simulink model "Robot_puma_system"  (R2018b)
settings: Solver=ode45  StartTime=0.0  StopTime=5  FixedStep=0.01  MaxStep=0.01  RelTol=1e-3
values from neighbouring files (symbols this model uses):
  AmpSat1 = 12    [CONSTANT.m]
  BackEMF1 = (12 - 38.1*0.2)/(40*2*pi/60)    (= 1.04564797611)    [CONSTANT.m]
  BackEMF2 = 0.32    [CONSTANT.m]
  BackEMF3 = 0.00091    [CONSTANT.m]
  CtlSat1 = 1024    [CONSTANT.m]
  Elec1d = [termL, termR1]    [CONSTANT.m]
  Elec1n = 1    [CONSTANT.m]
  Elec2d = [termL, termR2]    [CONSTANT.m]
  KP = [700 0 0 0 0 0; 0 670 0 0 0 0; 0 0 650 0 0 0; 0 0 0 400*5/1.5 0 0; 0 0 0 0 540*5/1.5 0; 0 0 0 0 0 210*5/1.5]    [CONSTANT.m]
  KV = [400 0 0 0 0 0; 0 470 0 0 0 0; 0 0 550 0 0 0; 0 0 0 370*5/1.5 0 0; 0 0 0 0 60*5/1.5 0; 0 0 0 0 0 180*5/1.5]    [CONSTANT.m]
  PWM_CONV_OTHER = 1.0/1024.0    (= 0.0009765625)    [CONSTANT.m]
  Starting_Pos = [0;3.1415926/5;3.1415926/6;3.1415926/10;3.1415926/7;3.1415926/2]    [CONSTANT.m]
  TConst1 = 1.207    [CONSTANT.m]
  TConst2 = 0.5324    [CONSTANT.m]
  TConst3 = 0.089240515    [CONSTANT.m]
settings Model: SimulationMode=accelerator  Creator=zhikai  LastModifiedBy=zhikai
settings SolverCC: AlgebraicLoopSolver=LineSearch
settings DataIOCC: SaveFinalState=on  SaveCompleteFinalSimState=on  SaveState=on

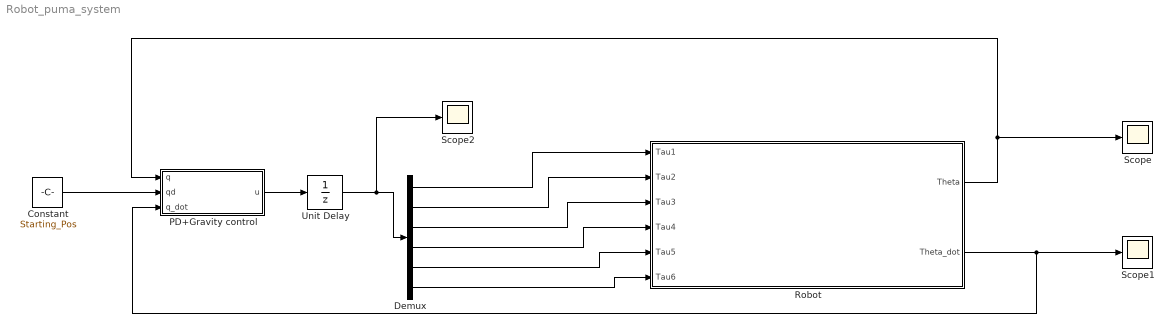
== system Robot_puma_system ==
  Constant : Constant  Value=Starting_Pos
  Demux : Demux  Outputs=6
  PD+Gravity control : Subsystem  TreatAsAtomicUnit=on
  Robot : Subsystem  TreatAsAtomicUnit=on
  Scope : Scope
  Scope1 : Scope
  Scope2 : Scope
  Unit Delay : UnitDelay  InitialCondition=[0;0;0;0;0;0]  SampleTime=-1
  wires:
  Demux/1 -> Robot/1(Tau1)
  Demux/2 -> Robot/2(Tau2)
  Constant/1 -> PD+Gravity control/2(qd)
  PD+Gravity control/1(u) -> Unit Delay/1
  Demux/3 -> Robot/3(Tau3)
  Demux/4 -> Robot/4(Tau4)
  Demux/5 -> Robot/5(Tau5)
  Demux/6 -> Robot/6(Tau6)
  Robot/2(Theta_dot) -> PD+Gravity control/3(q_dot), Scope1/1
  Robot/1(Theta) -> Scope/1, PD+Gravity control/1(q)
  Unit Delay/1 -> Scope2/1, Demux/1

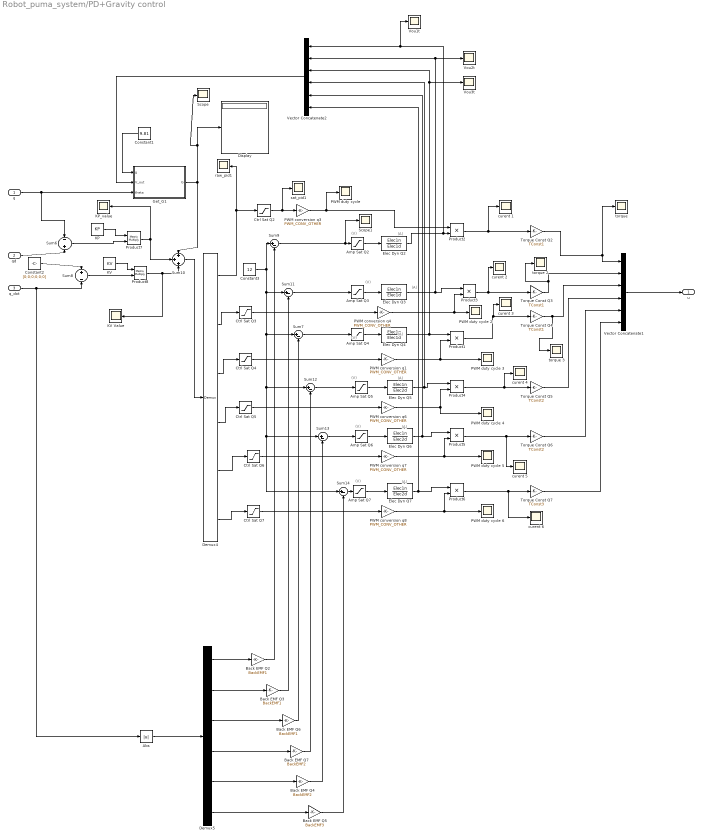
== system Robot_puma_system/PD+Gravity control ==
  note: (A)
  note: (V)
  note: (V)
  note: (A)
  note: (V)
  note: (A)
  note: (V)
  note: (A)
  note: (V)
  note: (A)
  note: (V)
  note: (A)
  q : Inport
  qd : Inport  Port=2
  q_dot : Inport  Port=3
  Abs : Abs
  Amp Sat Q{2..7} (6 alike) : Saturate  UpperLimit=AmpSat1  LowerLimit=0
  Back EMF Q2 : Gain  Gain=BackEMF1
  Back EMF Q3 : Gain  Gain=BackEMF1
  Back EMF Q4 : Gain  Gain=BackEMF2
  Back EMF Q5 : Gain  Gain=BackEMF3
  Back EMF Q6 : Gain  Gain=BackEMF1
  Back EMF Q7 : Gain  Gain=BackEMF2
  Constant1 : Constant  Value=9.81
  Constant2 : Constant  Value=[0;0;0;0;0;0]
  Constant3 : Constant  Value=12
  Ctrl Sat Q{2..7} (6 alike) : Saturate  UpperLimit=CtlSat1  LowerLimit=-CtlSat1
  Demux4 : Demux  Outputs=6
  Demux5 : Demux  Outputs=6
  Display : Display
      settings: Decimation=6
  Elec Dyn Q2 : TransferFcn  Numerator=Elec1n  Denominator=Elec1d
  Elec Dyn Q3 : TransferFcn  Numerator=Elec1n  Denominator=Elec1d
  Elec Dyn Q4 : TransferFcn  Numerator=Elec1n  Denominator=Elec1d
  Elec Dyn Q5 : TransferFcn  Numerator=Elec1n  Denominator=Elec2d
  Elec Dyn Q6 : TransferFcn  Numerator=Elec1n  Denominator=Elec2d
  Elec Dyn Q7 : TransferFcn  Numerator=Elec1n  Denominator=Elec2d
  Get_G1 : MATLAB Function  TreatAsAtomicUnit=on
  KP : Constant  Value=KP
  KP_value : Scope
  KV : Constant  Value=KV
  "KV Value " : Scope
  PWM conversion q{1,3..4,6..8} (6 alike) : Gain  Gain=PWM_CONV_OTHER
  PWM duty cycle : Scope
  PWM duty cycle {2..6} (5 alike) : Scope
  Product{1..6} (6 alike) : Product
  Product7 : Product  Multiplication=Matrix(*)
  Product8 : Product  Multiplication=Matrix(*)
  Scope : Scope
  Scope1 : Scope
  Sum10 : Sum  Inputs=+|+|+
  Sum{7,9,11..14} (6 alike) : Sum  Inputs=|+-
  Sum6 : Sum  Inputs=-|+
  Sum8 : Sum  Inputs=+|-
  Torque Const Q2 : Gain  Gain=TConst1
  Torque Const Q3 : Gain  Gain=TConst1
  Torque Const Q4 : Gain  Gain=TConst1
  Torque Const Q5 : Gain  Gain=TConst2
  Torque Const Q6 : Gain  Gain=TConst2
  Torque Const Q7 : Gain  Gain=TConst3
  Vector Concatenate1 : Concatenate  NumInputs=6
  Vector Concatenate2 : Concatenate  NumInputs=6
  Vou1t : Scope
  Vou2t : Scope
  Vou3t : Scope
  curent {1..6} (6 alike) : Scope
  raw_pid1 : Scope
  sat_pid1 : Scope
  "torque " : Scope
  torque 2 : Scope
  torque 3 : Scope
  u : Outport
  wires:
  Demux4/1 -> raw_pid1/1, Ctrl Sat Q2/1
  Constant2/1 -> Sum8/1
  Demux5/2 -> Back EMF Q3/1
  Sum10/1 -> Demux4/1
  PWM conversion q4/1 -> PWM duty cycle 2/1, Product3/2
  Torque Const Q3/1 -> torque 2/1, Vector Concatenate1/2
  Torque Const Q2/1 -> "torque "/1, Vector Concatenate1/1
  Demux5/1 -> Back EMF Q2/1
  q/1 -> Get_G1/3(theta), Sum6/1
  Demux4/2 -> Ctrl Sat Q3/1
  Elec Dyn Q2/1 -> Vou1t/1, Vector Concatenate2/1, Product2/2
  Vector Concatenate1/1 -> u/1
  Elec Dyn Q3/1 -> Vou2t/1, Vector Concatenate2/2, Product3/1
  Ctrl Sat Q2/1 -> sat_pid1/1, PWM conversion q3/1
  Sum6/1 -> Product7/2
  Ctrl Sat Q3/1 -> PWM conversion q4/1
  Product3/1 -> curent 2/1, Torque Const Q3/1
  qd/1 -> Sum6/2
  Product2/1 -> curent 1/1, Torque Const Q2/1
  q_dot/1 -> Sum8/2, Abs/1
  Amp Sat Q2/1 -> Elec Dyn Q2/1
  Sum9/1 -> Scope1/1, Amp Sat Q2/1
  Sum11/1 -> Amp Sat Q3/1
  Amp Sat Q3/1 -> Elec Dyn Q3/1
  Product8/1 -> "KV Value "/1, Sum10/3
  Product7/1 -> KP_value/1, Sum10/2
  Get_G1/1(G) -> Display/1, Scope/1, Sum10/1
  Elec Dyn Q4/1 -> Vector Concatenate2/3, Vou3t/1, Product1/1
  Sum7/1 -> Amp Sat Q4/1
  PWM conversion q1/1 -> Product1/2, PWM duty cycle 3/1
  Product1/1 -> curent 3/1, Torque Const Q4/1
  Amp Sat Q4/1 -> Elec Dyn Q4/1
  Torque Const Q4/1 -> torque 3/1, Vector Concatenate1/3
  Ctrl Sat Q4/1 -> PWM conversion q1/1
  Demux4/3 -> Ctrl Sat Q4/1
  Elec Dyn Q5/1 -> Vector Concatenate2/4, Product4/1
  Sum12/1 -> Amp Sat Q5/1
  PWM conversion q6/1 -> PWM duty cycle 4/1, Product4/2
  Product4/1 -> curent 4/1, Torque Const Q5/1
  Amp Sat Q5/1 -> Elec Dyn Q5/1
  Torque Const Q5/1 -> Vector Concatenate1/4
  Ctrl Sat Q5/1 -> PWM conversion q6/1
  Demux4/4 -> Ctrl Sat Q5/1
  Elec Dyn Q6/1 -> Vector Concatenate2/5, Product5/1
  Sum13/1 -> Amp Sat Q6/1
  PWM conversion q7/1 -> PWM duty cycle 5/1, Product5/2
  Product5/1 -> curent 5/1, Torque Const Q6/1
  Amp Sat Q6/1 -> Elec Dyn Q6/1
  Torque Const Q6/1 -> Vector Concatenate1/5
  Ctrl Sat Q6/1 -> PWM conversion q7/1
  Elec Dyn Q7/1 -> Vector Concatenate2/6, Product6/1
  Sum14/1 -> Amp Sat Q7/1
  PWM conversion q8/1 -> PWM duty cycle 6/1, Product6/2
  Product6/1 -> curent 6/1, Torque Const Q7/1
  Constant3/1 -> Sum11/1, Sum7/1, Sum14/1, Sum13/1, Sum12/1, Sum9/1
  Amp Sat Q7/1 -> Elec Dyn Q7/1
  Torque Const Q7/1 -> Vector Concatenate1/6
  Ctrl Sat Q7/1 -> PWM conversion q8/1
  Demux4/6 -> Ctrl Sat Q7/1
  Demux5/5 -> Back EMF Q4/1
  Demux5/6 -> Back EMF Q5/1
  Demux5/3 -> Back EMF Q6/1
  Demux5/4 -> Back EMF Q7/1
  Back EMF Q2/1 -> Sum9/2
  Back EMF Q3/1 -> Sum11/2
  Back EMF Q6/1 -> Sum7/2
  Back EMF Q7/1 -> Sum12/2
  Back EMF Q4/1 -> Sum13/2
  Back EMF Q5/1 -> Sum14/2
  Vector Concatenate2/1 -> Get_G1/2(V_out)
  Constant1/1 -> Get_G1/1(g)
  Demux4/5 -> Ctrl Sat Q6/1
  PWM conversion q3/1 -> Product2/1, PWM duty cycle/1
  KP/1 -> Product7/1
  KV/1 -> Product8/1
  Sum8/1 -> Product8/2
  Abs/1 -> Demux5/1

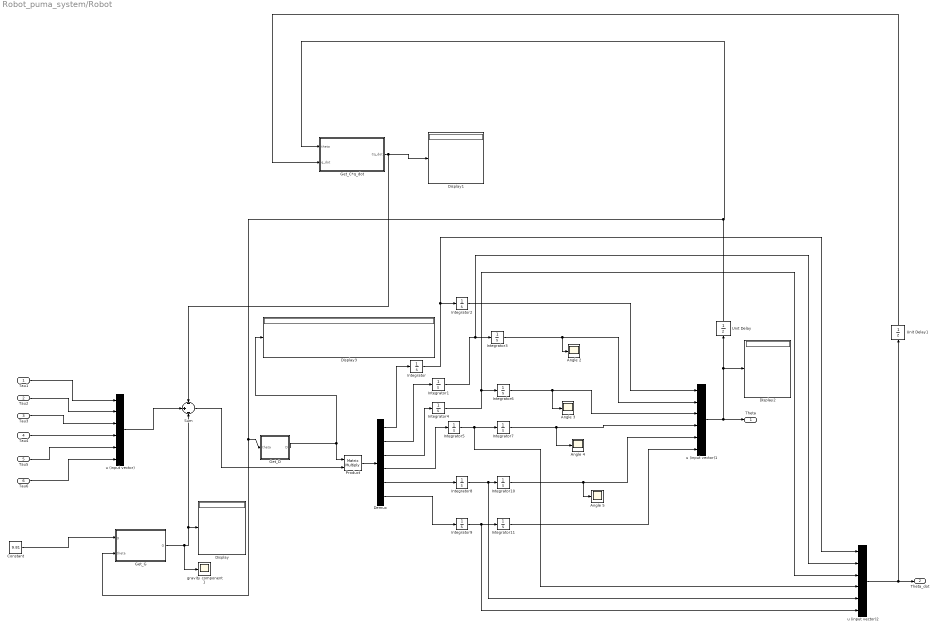
== system Robot_puma_system/Robot ==
  Tau1 : Inport
  Tau2 : Inport  Port=2
  Tau3 : Inport  Port=3
  Tau4 : Inport  Port=4
  Tau5 : Inport  Port=5
  Tau6 : Inport  Port=6
  Angle {2..5} (4 alike) : Scope
  Constant : Constant  Value=9.81
  Demux : Demux  Outputs=6
  Display{,1..3} (4 alike) : Display
      Display settings: Decimation=6
      Display1 settings: Decimation=6
      Display2 settings: Decimation=6
      Display3 settings: Decimation=36
  Get_C*q_dot : MATLAB Function  TreatAsAtomicUnit=on
  Get_D : MATLAB Function  TreatAsAtomicUnit=on
  Get_G : MATLAB Function  TreatAsAtomicUnit=on
  Integrator{,1,3..11} (11 alike) : Integrator
  Integrator2 : Integrator  InitialCondition=-pi/2
  Product : Product  Multiplication=Matrix(*)
  Sum : Sum  Inputs=-|+|-
  Unit Delay : UnitDelay  InitialCondition=[-pi/2;0;0;0;0;0]  SampleTime=-1
  Unit Delay1 : UnitDelay  InitialCondition=[0;0;0;0;0;0]  SampleTime=-1
  gravity component 1 : Scope
  u (input vector) : Concatenate  NumInputs=6
  u (input vector)1 : Concatenate  NumInputs=6
  u (input vector)2 : Concatenate  NumInputs=6
  Theta : Outport
  Theta_dot : Outport  Port=2
  wires:
  Tau2/1 -> u (input vector)/2
  Get_C*q_dot/1(Cq_dot) -> Display1/1, Sum/1
  Demux/1 -> Integrator/1
  Tau1/1 -> u (input vector)/1
  Sum/1 -> Product/2
  Integrator1/1 -> Integrator3/1, u (input vector)2/2
  Get_G/1(G) -> gravity component 1/1, Sum/3, Display/1
  u (input vector)/1 -> Sum/2
  Demux/2 -> Integrator1/1
  Integrator/1 -> Integrator2/1, u (input vector)2/1
  Tau3/1 -> u (input vector)/3
  Tau4/1 -> u (input vector)/4
  Tau6/1 -> u (input vector)/6
  Tau5/1 -> u (input vector)/5
  Integrator4/1 -> Integrator6/1, u (input vector)2/3
  Demux/3 -> Integrator4/1
  Demux/4 -> Integrator5/1
  Integrator8/1 -> u (input vector)2/5, Integrator10/1
  Integrator9/1 -> u (input vector)2/6, Integrator11/1
  Demux/5 -> Integrator8/1
  Demux/6 -> Integrator9/1
  Integrator2/1 -> u (input vector)1/1
  Integrator3/1 -> Angle 2/1, u (input vector)1/2
  Integrator6/1 -> Angle 3/1, u (input vector)1/3
  Integrator7/1 -> Angle 4/1, u (input vector)1/4
  Integrator10/1 -> Angle 5/1, u (input vector)1/5
  Integrator11/1 -> u (input vector)1/6
  Integrator5/1 -> u (input vector)2/4, Integrator7/1
  Constant/1 -> Get_G/1(g)
  Product/1 -> Demux/1
  u (input vector)1/1 -> Unit Delay/1, Display2/1, Theta/1
  u (input vector)2/1 -> Unit Delay1/1, Theta_dot/1
  Unit Delay/1 -> Get_C*q_dot/1(theta), Get_G/2(theta), Get_D/1(theta)
  Unit Delay1/1 -> Get_C*q_dot/2(q_dot)
  Get_D/1(D) -> Product/1, Display3/1

== matlab function Robot_puma_system/Robot/Get_D ==
  data: theta input; D output size=[6,6]
function D = fcn(theta)
   D = zeros(6,6);
   coder.extrinsic('D_gen');
   D_temp = D_gen(theta);
   D = inv(D_temp);
   %D = D + J_rotor;
end

== matlab function Robot_puma_system/Robot/Get_C*q_dot ==
  data: theta input; Cq_dot output size=[6,1]; q_dot input
function Cq_dot = Get_Cq_dot(theta,   q_dot)
    Cq_dot = zeros(6,1);
    eml.extrinsic('C_gen');
    C_temp = C_gen(theta, q_dot);
    Cq_dot = C_temp;
end

== matlab function Robot_puma_system/Robot/Get_G ==
  data: g input; G output size=[6,1]; theta input
function G = Get_G( g, theta)
    G = zeros(6,1);
    eml.extrinsic('G_gen');
    G = G_gen(g,theta);
end

== matlab function Robot_puma_system/PD+Gravity control/Get_G1 ==
  data: g input; V_out input size=[6,1]; theta input; G output
function G = Get_G( g, V_out, theta)
    G = zeros(6,1);
    G_temp = zeros(6,1);
    Torque_const1 = 1.307;
    Torque_const2 = 0.5324;
    Torque_const3 = 0.089240515;
    %eml.extrinsic
    eml.extrinsic('G_gen');
    G_temp = G_gen(g,theta);
    %G = [((m1+m2)*l1*9.81*cos(theta1) + m2*l2*9.81*cos(theta1 + theta2))/V_out1; m2*l2*9.81*cos(theta1 + theta2)/V_out2];
    for i_G = 1:6
        if (G_temp(i_G) ~= 0)
            %G_temp(i_G) = 0.000001;
            G_temp(i_G) = G_temp(i_G)/V_out(i_G);
        end
        %G_temp(i_G) = G_temp(i_G)/V_out(i_G);
        if (i_G < 3)
            G_temp(i_G) = G_temp(i_G)/Torque_const1;
        
        elseif (i_G < 5)
            G_temp(i_G) = G_temp(i_G)/Torque_const2;
           
        else
            G_temp(i_G) = G_temp(i_G)/Torque_const3;
        end
    end
    G_temp = G_temp.*(1024);
    G = G_temp;
end
